simulink model "SIMU"  (R2013a)
settings: Solver=ode45  StartTime=0.0  StopTime=10.0  RelTol=1e-3
values from neighbouring files (symbols this model uses):
  C = 0.1e-4    (= 1e-05)    [FT_primer_orden.m]    (also in SIMULINK.mat = 0.1; clase1.m = 5e-06; ejem_ss2tf.m = [ -0.1241    1.4090; prac_00.mat = [12 9 6 12 18])
  L = 1    [SIMULINK.mat]    (also in clase1.m = 0.002; prac_00.mat = [-24 9 -4 16 36]; pract.mat)
  R = 1000    [FT_primer_orden.m]    (also in SIMULINK.mat = 1; clase1.m; prac_00.mat = [1  1  1  1; 1  1  1  1; 1  1  1  1]; pract.mat = 1)
settings Model: Creator=Administrador  LastModifiedBy=Administrador

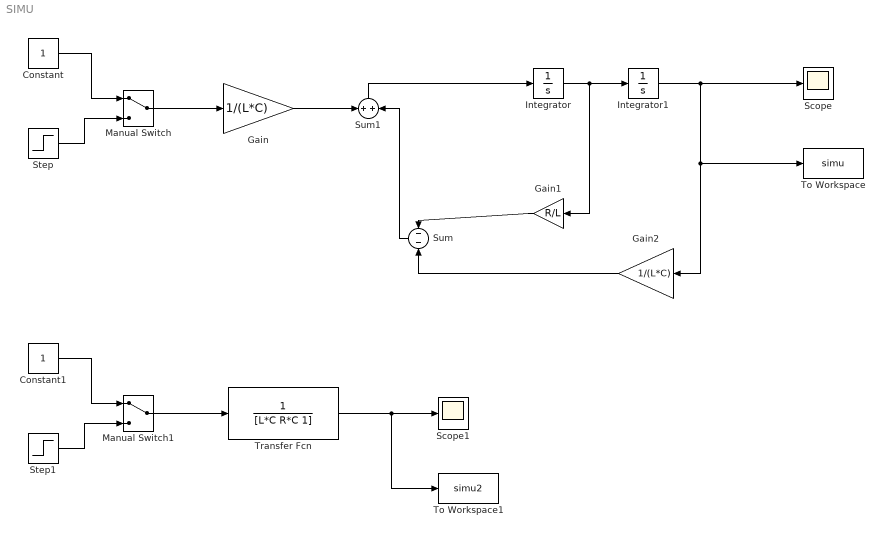
== system SIMU ==
  Constant : Constant
  Constant1 : Constant
  Gain : Gain  Gain=1/(L*C)
  Gain1 : Gain  Gain=R/L
  Gain2 : Gain  Gain=1/(L*C)
  Integrator : Integrator
  Integrator1 : Integrator
  Manual Switch : ManualSwitch
  Manual Switch1 : ManualSwitch
  Scope : Scope
  Scope1 : Scope
  Step : Step  SampleTime=0
  Step1 : Step  SampleTime=0
  Sum : Sum  Inputs=--
  Sum1 : Sum
  To Workspace : ToWorkspace  VariableName=simu  SampleTime=-1
  To Workspace1 : ToWorkspace  VariableName=simu2  SampleTime=-1
  Transfer Fcn : TransferFcn  Denominator=[L*C R*C 1]
  wires:
  Constant/1 -> Manual Switch/1
  Step/1 -> Manual Switch/2
  Constant1/1 -> Manual Switch1/1
  Step1/1 -> Manual Switch1/2
  Manual Switch/1 -> Gain/1
  Integrator/1 -> Gain1/1, Integrator1/1
  Integrator1/1 -> To Workspace/1, Gain2/1, Scope/1
  Manual Switch1/1 -> Transfer Fcn/1
  Gain1/1 -> Sum/1
  Gain2/1 -> Sum/2
  Sum/1 -> Sum1/2
  Gain/1 -> Sum1/1
  Sum1/1 -> Integrator/1
  Transfer Fcn/1 -> To Workspace1/1, Scope1/1
